simulink model "hx_sim"  (R2017b)
settings: Solver=ode23tb  StartTime=0.0  StopTime=tEndSimul  MaxStep=0.1  RelTol=5e-6
values from neighbouring files (symbols this model uses):
  dnDt_in = 1e-2    (= 0.01)    [hx.m]
  dnDt_out_liq = 1e-2    (= 0.01)    [hx.m]
  dnDt_out_vap = 1e-2    (= 0.01)    [hx.m]
  fluid = nh3_v4    [hx.m]
  Nhx_init = 100    [hx.m]
  q = 1e2    (= 100)    [hx.m]
  T_dnDt_in_C = 50    [hx.m]
  tEnd_dnDt_in = tStart_dnDt_in + 10 * c.min_to_sec    [hx.m]
  tEnd_dnDt_out_liq = tStart_dnDt_out_liq + 10 * c.min_to_sec    [hx.m]
  tEnd_dnDt_out_vap = tStart_dnDt_out_vap + 10 * c.min_to_sec    [hx.m]
  tEnd_q = tStart_q + 10 * c.min_to_sec    [hx.m]
  Thx_init = c.C_to_K(25)    [hx.m]
  tStart_dnDt_in = tEnd_q + 10 * c.min_to_sec    [hx.m]
  tStart_dnDt_out_liq = tEnd_dnDt_out_vap + 10 * c.min_to_sec    [hx.m]
  tStart_dnDt_out_vap = tEnd_dnDt_in + 10 * c.min_to_sec    [hx.m]
  tStart_q = 5 * c.min_to_sec    [hx.m]
  Vhx = 0.01    [hx.m]
libraries: thermochemical x20
settings Model: Creator=ferru  LastModifiedBy=fferrucc
settings SolverCC: AlgebraicLoopSolver=LineSearch

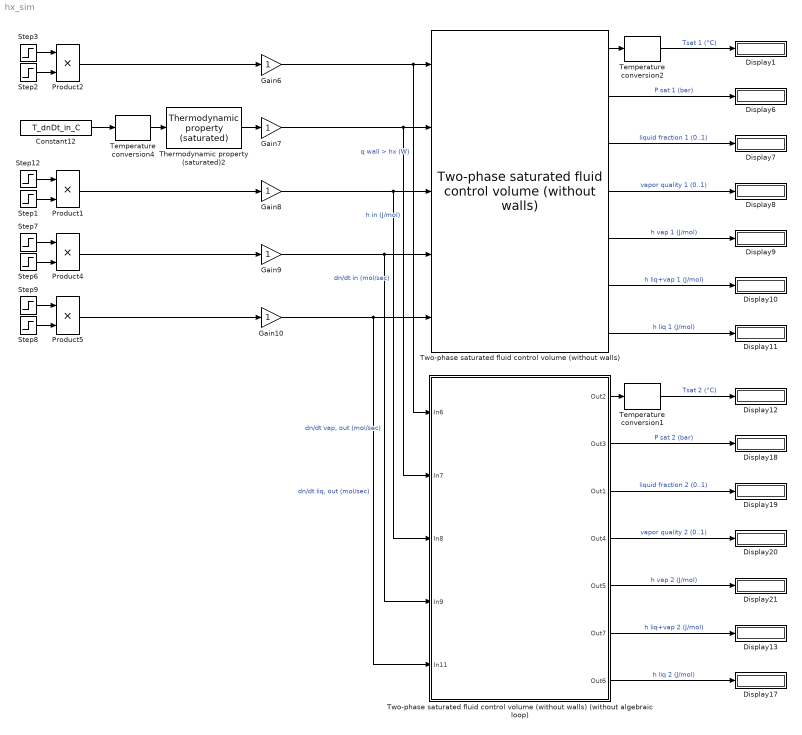
== system hx_sim ==
  Constant12 : Constant  Value=T_dnDt_in_C
  Display{1,6..13,17..21} (14 alike) : Display
  Gain{6..10} (5 alike) : Gain
  Product{1..2,4..5} (4 alike) : Product
  Step1 : Step  Time=tEnd_dnDt_in  Before=1  After=0  SampleTime=0
  Step12 : Step  Time=tStart_dnDt_in  After=dnDt_in  SampleTime=0
  Step2 : Step  Time=tEnd_q  Before=1  After=0  SampleTime=0
  Step3 : Step  Time=tStart_q  After=q  SampleTime=0
  Step6 : Step  Time=tEnd_dnDt_out_vap  Before=1  After=0  SampleTime=0
  Step7 : Step  Time=tStart_dnDt_out_vap  After=dnDt_out_vap  SampleTime=0
  Step8 : Step  Time=tEnd_dnDt_out_liq  Before=1  After=0  SampleTime=0
  Step9 : Step  Time=tStart_dnDt_out_liq  After=dnDt_out_liq  SampleTime=0
  Temperature conversion1 : thermochemical/Conversions/Temperature conversion  sel=K --> °C
      settings: SourceProductName=@ Thermochemical
  Temperature conversion2 : thermochemical/Conversions/Temperature conversion  sel=K --> °C
      settings: SourceProductName=@ Thermochemical
  Temperature conversion4 : thermochemical/Conversions/Temperature conversion  sel=°C --> K
      settings: SourceProductName=@ Thermochemical
  Thermodynamic property (saturated)2 : thermochemical/Thermodynamic fluid properties/Thermodynamic  property (saturated)  sel=h(T) vap. (J/mol)  fluid=fluid  lookup1D_BreakPoint1=fluid.sat.T  lookup1D_Data=fluid.sat.vap.h_molar
      settings: SourceProductName=@ Thermochemical
  Two-phase saturated fluid control volume (without walls) : thermochemical/Control volumes/Two-phase saturated fluid control volume (without walls)  N_init=Nhx_init  T_init=Thx_init  fluid=fluid  V=Vhx
      settings: SourceProductName=@ Thermochemical
  Two-phase saturated fluid control volume (without walls) (without algebraic loop) : Subsystem  AncestorBlock=|  mask(volume_control_saturated){N_init=Nhx_init, T_init=Thx_init, fluid=fluid, V=Vhx}
      | thermochemical/Control volumes/Two-phase saturated fluid
      | control volume (without walls)
      | (without algebraic loop)
      mask prompts: N_init "Initial number of mols inside the control volume (mol)"; T_init "Fluid initial temperature (K)"; fluid "Fluid (structure data type)"; V "Volume (m3)"
      mask help:
      | This block models a volume control that contains a fluid always in its saturation state.
      |
      | The model can work as a condenser or as an evaporator:
      | • Condenser: connect the output 'h liq (J/mol)' to the input 'h out (sat) (J/mol)'
      | • Evaporator: connect the output 'h vap (J/mol)' to the input 'h out (sat) (J/mol)'
      |
      | The ratio between the two phases is given by two outputs:
      | 1) volumetric liquid fraction: liquid volume/total volume (0..1)
      | 2) vapor quality (e.g. zero: 100% liquid, one: 100% vapor).
      |
      | Note 2: the model is not prepared to work in the non-saturation state of the fluid (e.g. superheated gas or supercooled liquid). This means that both the liquid fraction and the vapor quality are strictly constrained in the (0..1) open range. The simulation will stop if these constrains are violated.
      mask init:
      | c = conversion_factors();
      mask DialogControl Container3 Prompt: Initial state
      mask DialogControl Container4 Prompt: Other parameters
  wires:
  Step12/1 -> Product1/1
  Step1/1 -> Product1/2
  Constant12/1 -> Temperature conversion4/1
  Temperature conversion4/1 -> Thermodynamic property (saturated)2/1
  Temperature conversion2/1 -> Display1/1  "Tsat 1 (°C)"
  Two-phase saturated fluid control volume (without walls)/1 -> Temperature conversion2/1
  Gain6/1 -> Two-phase saturated fluid control volume (without walls) (without algebraic loop)/1(In6), Two-phase saturated fluid control volume (without walls)/1  "q wall > hx (W)"
  Gain7/1 -> Two-phase saturated fluid control volume (without walls) (without algebraic loop)/2(In7), Two-phase saturated fluid control volume (without walls)/2  "h in (J/mol)"
  Gain8/1 -> Two-phase saturated fluid control volume (without walls) (without algebraic loop)/3(In8), Two-phase saturated fluid control volume (without walls)/3  "dn/dt in (mol/sec)"
  Gain9/1 -> Two-phase saturated fluid control volume (without walls) (without algebraic loop)/4(In9), Two-phase saturated fluid control volume (without walls)/4  "dn/dt vap, out (mol/sec)"
  Gain10/1 -> Two-phase saturated fluid control volume (without walls) (without algebraic loop)/5(In11), Two-phase saturated fluid control volume (without walls)/5  "dn/dt liq, out (mol/sec)"
  Two-phase saturated fluid control volume (without walls)/2 -> Display6/1  "P sat 1 (bar)"
  Two-phase saturated fluid control volume (without walls)/3 -> Display7/1  "liquid fraction 1 (0..1)"
  Two-phase saturated fluid control volume (without walls)/4 -> Display8/1  "vapor quality 1 (0..1)"
  Two-phase saturated fluid control volume (without walls)/5 -> Display9/1  "h vap 1 (J/mol)"
  Two-phase saturated fluid control volume (without walls)/6 -> Display10/1  "h liq+vap 1 (J/mol)"
  Two-phase saturated fluid control volume (without walls)/7 -> Display11/1  "h liq 1 (J/mol)"
  Two-phase saturated fluid control volume (without walls) (without algebraic loop)/7(Out6) -> Display17/1  "h liq 2 (J/mol)"
  Two-phase saturated fluid control volume (without walls) (without algebraic loop)/6(Out7) -> Display13/1  "h liq+vap 2 (J/mol)"
  Two-phase saturated fluid control volume (without walls) (without algebraic loop)/5(Out5) -> Display21/1  "h vap 2 (J/mol)"
  Two-phase saturated fluid control volume (without walls) (without algebraic loop)/4(Out4) -> Display20/1  "vapor quality 2 (0..1)"
  Two-phase saturated fluid control volume (without walls) (without algebraic loop)/3(Out1) -> Display19/1  "liquid fraction 2 (0..1)"
  Two-phase saturated fluid control volume (without walls) (without algebraic loop)/2(Out3) -> Display18/1  "P sat 2 (bar)"
  Two-phase saturated fluid control volume (without walls) (without algebraic loop)/1(Out2) -> Temperature conversion1/1
  Temperature conversion1/1 -> Display12/1  "Tsat 2 (°C)"
  Step2/1 -> Product2/2
  Step3/1 -> Product2/1
  Product2/1 -> Gain6/1
  Thermodynamic property (saturated)2/1 -> Gain7/1
  Product1/1 -> Gain8/1
  Product4/1 -> Gain9/1
  Step6/1 -> Product4/2
  Step7/1 -> Product4/1
  Step9/1 -> Product5/1
  Step8/1 -> Product5/2
  Product5/1 -> Gain10/1

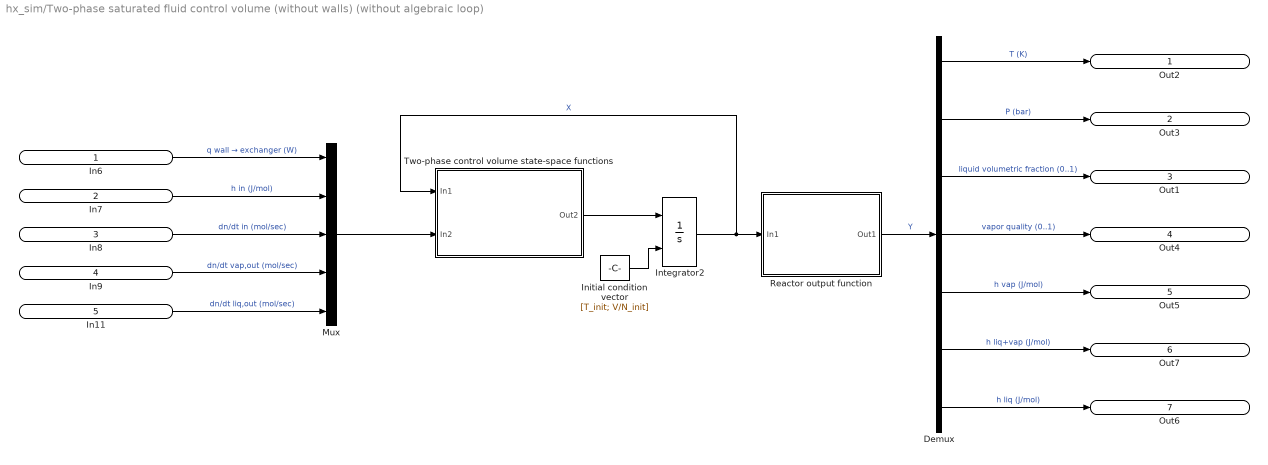
== system hx_sim/Two-phase saturated fluid control volume (without walls) (without algebraic loop) ==
  In6 : Inport
  In7 : Inport  Port=2
  In8 : Inport  Port=3
  In9 : Inport  Port=4
  In11 : Inport  Port=5
  Demux : Demux  Outputs=7
  Initial condition vector : Constant  Value=[T_init; V/N_init]
  Integrator2 : Integrator  InitialConditionSource=external
  Mux : Mux  Inputs=5
  Reactor output function : Subsystem
  Two-phase control volume state-space functions : Subsystem
  Out2 : Outport
  Out3 : Outport  Port=2
  Out1 : Outport  Port=3
  Out4 : Outport  Port=4
  Out5 : Outport  Port=5
  Out7 : Outport  Port=6
  Out6 : Outport  Port=7
  wires:
  Integrator2/1 -> Two-phase control volume state-space functions/1(In1), Reactor output function/1(In1)  "X"
  Initial condition vector/1 -> Integrator2/2
  Two-phase control volume state-space functions/1(Out2) -> Integrator2/1
  Mux/1 -> Two-phase control volume state-space functions/2(In2)
  Reactor output function/1(Out1) -> Demux/1  "Y"
  Demux/7 -> Out6/1  "h liq (J/mol)"
  Demux/2 -> Out3/1  "P (bar)"
  Demux/6 -> Out7/1  "h liq+vap (J/mol)"
  Demux/5 -> Out5/1  "h vap (J/mol)"
  Demux/4 -> Out4/1  "vapor quality (0..1)"
  Demux/1 -> Out2/1  "T (K)"
  Demux/3 -> Out1/1  "liquid volumetric fraction (0..1)"
  In6/1 -> Mux/1  "q wall → exchanger (W)"
  In11/1 -> Mux/5  "dn/dt liq,out (mol/sec)"
  In8/1 -> Mux/3  "dn/dt in (mol/sec)"
  In7/1 -> Mux/2  "h in (J/mol)"
  In9/1 -> Mux/4  "dn/dt vap,out (mol/sec)"

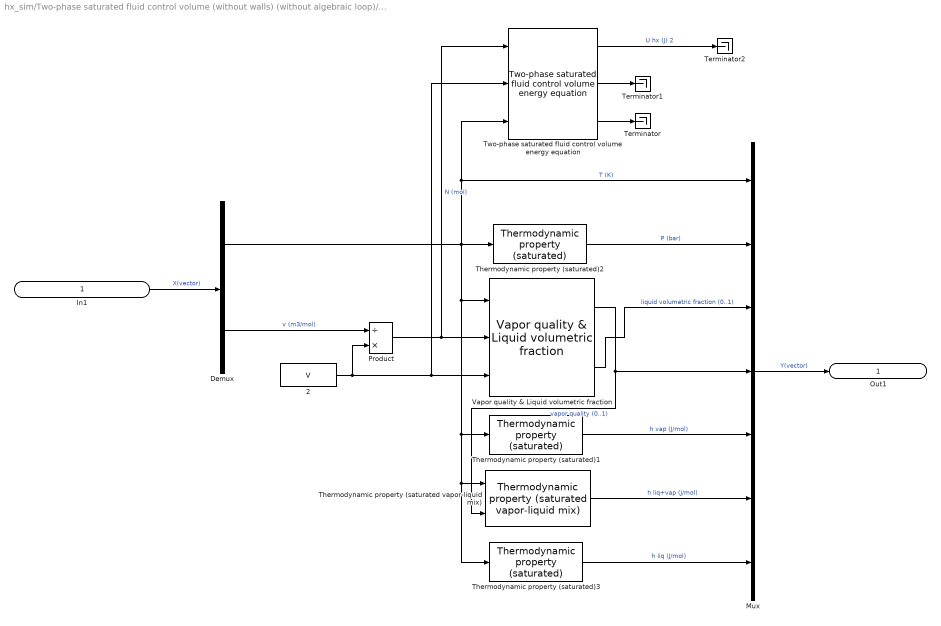
== system hx_sim/Two-phase saturated fluid control volume (without walls) (without algebraic loop)/Reactor output function ==
  In1 : Inport
  2 : Constant  Value=V
  Demux : Demux  Outputs=2
  Mux : Mux  Inputs=7
  Product : Product  Inputs=/*
  Terminator : Terminator
  Terminator1 : Terminator
  Terminator2 : Terminator
  Thermodynamic property (saturated)1 : thermochemical/Thermodynamic fluid properties/Thermodynamic  property (saturated)  sel=h(T) vap. (J/mol)  fluid=fluid  lookup1D_BreakPoint1=fluid.sat.T  lookup1D_Data=fluid.sat.vap.h_molar
      settings: SourceProductName=@ Thermochemical
  Thermodynamic property (saturated)2 : thermochemical/Thermodynamic fluid properties/Thermodynamic  property (saturated)  sel=P(T) (bar)  fluid=fluid  lookup1D_BreakPoint1=fluid.sat.T  lookup1D_Data=fluid.sat.Psat
      settings: SourceProductName=@ Thermochemical
  Thermodynamic property (saturated)3 : thermochemical/Thermodynamic fluid properties/Thermodynamic  property (saturated)  sel=h(T) liq. (J/mol)  fluid=fluid  lookup1D_BreakPoint1=fluid.sat.T  lookup1D_Data=fluid.sat.liq.h_molar
      settings: SourceProductName=@ Thermochemical
  Thermodynamic property (saturated vapor-liquid mix) : thermochemical/Thermodynamic fluid properties/Thermodynamic property  (saturated vapor-liquid mix)  sel=h(T) (J/mol)  fluid=fluid  lookup1D_BreakPoint=0  lookup1D_Data1=fluid.sat.liq.h_molar  lookup1D_Data2=fluid.sat.vap.h_molar
      settings: SourceProductName=@ Thermochemical
  Two-phase saturated fluid control volume energy equation : thermochemical/Control volumes/Two-phase saturated fluid control volume energy equation  fluid=fluid
      settings: SourceProductName=@ Thermochemical
  Vapor quality & Liquid volumetric fraction : thermochemical/Thermodynamic fluid properties/Vapor quality & Liquid  volumetric fraction  fluid=fluid
      settings: SourceProductName=@ Thermochemical
  Out1 : Outport
  wires:
  Demux/1 -> Thermodynamic property (saturated)3/1, Thermodynamic property (saturated vapor-liquid mix)/1, Thermodynamic property (saturated)1/1, Vapor quality & Liquid volumetric fraction/1, Two-phase saturated fluid control volume energy equation/3, Mux/1, Thermodynamic property (saturated)2/1  "T (K)"
  Demux/2 -> Product/1  "v (m3/mol)"
  Mux/1 -> Out1/1  "Y(vector)"
  In1/1 -> Demux/1  "X(vector)"
  Vapor quality & Liquid volumetric fraction/1 -> Thermodynamic property (saturated vapor-liquid mix)/2, Mux/4  "vapor quality (0..1)"
  Thermodynamic property (saturated)1/1 -> Mux/5  "h vap (J/mol)"
  Vapor quality & Liquid volumetric fraction/2 -> Mux/3  "liquid volumetric fraction (0..1)"
  Thermodynamic property (saturated vapor-liquid mix)/1 -> Mux/6  "h liq+vap (J/mol)"
  Thermodynamic property (saturated)2/1 -> Mux/2  "P (bar)"
  Thermodynamic property (saturated)3/1 -> Mux/7  "h liq (J/mol)"
  Product/1 -> Vapor quality & Liquid volumetric fraction/2, Two-phase saturated fluid control volume energy equation/1  "N (mol)"
  2/1 -> Two-phase saturated fluid control volume energy equation/2, Vapor quality & Liquid volumetric fraction/3, Product/2
  Two-phase saturated fluid control volume energy equation/3 -> Terminator/1
  Two-phase saturated fluid control volume energy equation/2 -> Terminator1/1
  Two-phase saturated fluid control volume energy equation/1 -> Terminator2/1  "U hx (J) 2"

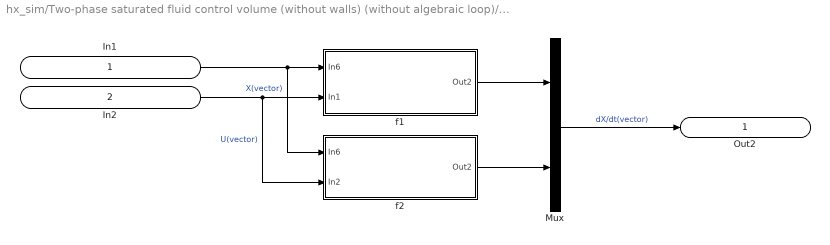
== system hx_sim/Two-phase saturated fluid control volume (without walls) (without algebraic loop)/Two-phase control volume state-space functions ==
  In1 : Inport
  In2 : Inport  Port=2
  Mux : Mux  Inputs=2
  f1 : Subsystem
  f2 : Subsystem
  Out2 : Outport
  wires:
  In2/1 -> f2/2(In2), f1/2(In1)  "U(vector)"
  In1/1 -> f2/1(In6), f1/1(In6)  "X(vector)"
  Mux/1 -> Out2/1  "dX/dt(vector)"
  f1/1(Out2) -> Mux/1
  f2/1(Out2) -> Mux/2

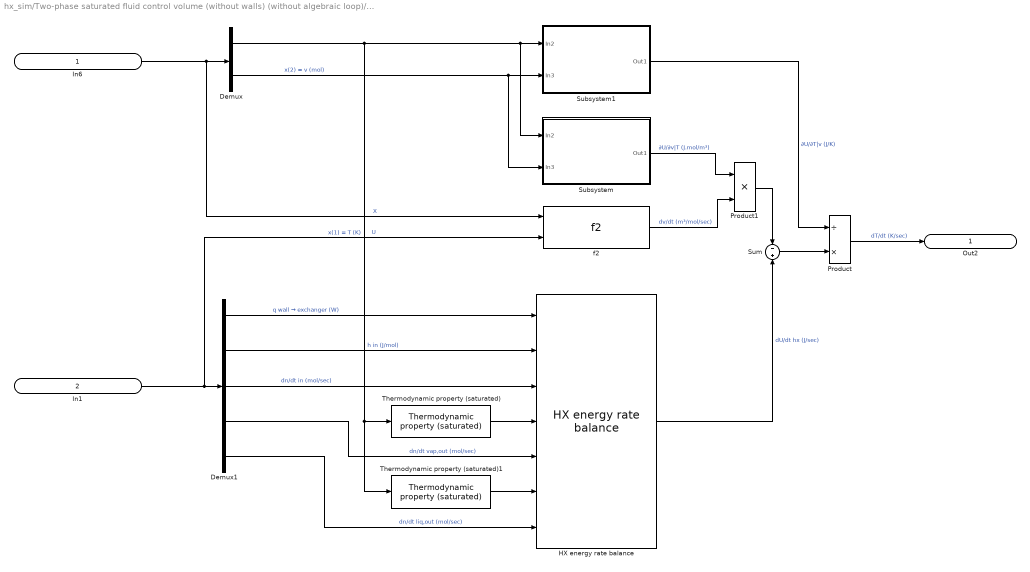
== system hx_sim/Two-phase saturated fluid control volume (without walls) (without algebraic loop)/Two-phase control volume state-space functions/f1 ==
  In6 : Inport
  In1 : Inport  Port=2
  Demux : Demux  Outputs=2
  Demux1 : Demux  Outputs=5
  HX energy rate balance : thermochemical/Control volumes/Two-phase saturated fluid control volume (without walls)/Internal energy differential equation/HX energy rate balance
      settings: SourceProductName=@ Thermochemical
  Product : Product  Inputs=/*
  Product1 : Product  Inputs=**
  Subsystem : Subsystem
  Subsystem1 : Subsystem
  Sum : Sum  Inputs=-+
  Thermodynamic property (saturated) : thermochemical/Thermodynamic fluid properties/Thermodynamic  property (saturated)  sel=h(T) vap. (J/mol)  fluid=fluid  lookup1D_BreakPoint1=fluid.sat.T  lookup1D_Data=fluid.sat.vap.h_molar
      settings: SourceProductName=@ Thermochemical
  Thermodynamic property (saturated)1 : thermochemical/Thermodynamic fluid properties/Thermodynamic  property (saturated)  sel=h(T) liq. (J/mol)  fluid=fluid  lookup1D_BreakPoint1=fluid.sat.T  lookup1D_Data=fluid.sat.liq.h_molar
      settings: SourceProductName=@ Thermochemical
  f2 : thermochemical/Control volumes/Two-phase saturated fluid control volume (without walls) (without algebraic loop)/Two-phase control volume state-space functions/f2
      settings: SourceProductName=@ Thermochemical
  Out2 : Outport
  wires:
  Product/1 -> Out2/1  "dT/dt (K/sec)"
  Demux/2 -> Subsystem/2(In3), Subsystem1/2(In3)  "x(2) = v (mol)"
  In6/1 -> f2/1, Demux/1  "X"
  In1/1 -> f2/2, Demux1/1  "U"
  Demux/1 -> Thermodynamic property (saturated)1/1, Thermodynamic property (saturated)/1, Subsystem/1(In2), Subsystem1/1(In2)  "x(1) = T (K)"
  HX energy rate balance/1 -> Sum/2  "dU/dt hx (J/sec)"
  Subsystem/1(Out1) -> Product1/1  "∂U/∂v|T (J.mol/m³)"
  Subsystem1/1(Out1) -> Product/1  "∂U/∂T|v (J/K)"
  f2/1 -> Product1/2  "dv/dt (m³/mol/sec)"
  Sum/1 -> Product/2
  Product1/1 -> Sum/1
  Demux1/1 -> HX energy rate balance/1  "q wall → exchanger (W)"
  Demux1/3 -> HX energy rate balance/3  "dn/dt in (mol/sec)"
  Demux1/4 -> HX energy rate balance/5  "dn/dt vap,out (mol/sec)"
  Demux1/2 -> HX energy rate balance/2  "h in (J/mol)"
  Demux1/5 -> HX energy rate balance/7  "dn/dt liq,out (mol/sec)"
  Thermodynamic property (saturated)/1 -> HX energy rate balance/4
  Thermodynamic property (saturated)1/1 -> HX energy rate balance/6

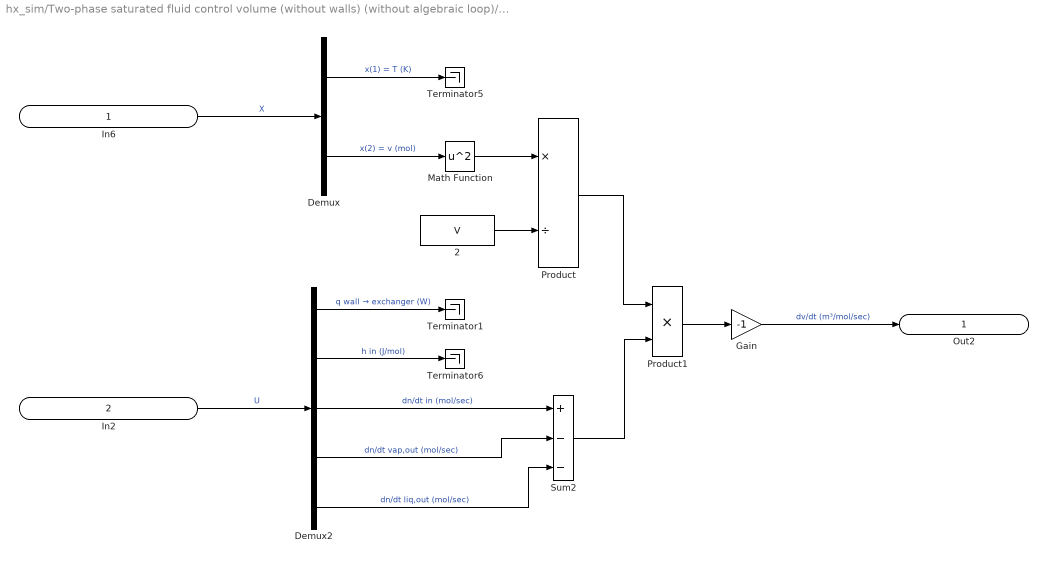
== system hx_sim/Two-phase saturated fluid control volume (without walls) (without algebraic loop)/Two-phase control volume state-space functions/f2 ==
  In6 : Inport
  In2 : Inport  Port=2
  2 : Constant  Value=V
  Demux : Demux  Outputs=2
  Demux2 : Demux  Outputs=5
  Gain : Gain  Gain=-1
  Math Function : Math  Operator=square  SaturateOnIntegerOverflow=on
  Product : Product  Inputs=*/
  Product1 : Product  Inputs=**
  Sum2 : Sum  Inputs=+--
  Terminator1 : Terminator
  Terminator5 : Terminator
  Terminator6 : Terminator
  Out2 : Outport
  wires:
  Demux/1 -> Terminator5/1  "x(1) = T (K)"
  In6/1 -> Demux/1  "X"
  Product1/1 -> Gain/1
  Demux/2 -> Math Function/1  "x(2) = v (mol)"
  Sum2/1 -> Product1/2
  Math Function/1 -> Product/1
  2/1 -> Product/2
  Product/1 -> Product1/1
  Demux2/2 -> Terminator6/1  "h in (J/mol)"
  Demux2/3 -> Sum2/1  "dn/dt in (mol/sec)"
  Demux2/1 -> Terminator1/1  "q wall → exchanger (W)"
  Demux2/5 -> Sum2/3  "dn/dt liq,out (mol/sec)"
  Demux2/4 -> Sum2/2  "dn/dt vap,out (mol/sec)"
  In2/1 -> Demux2/1  "U"
  Gain/1 -> Out2/1  "dv/dt (m³/mol/sec)"

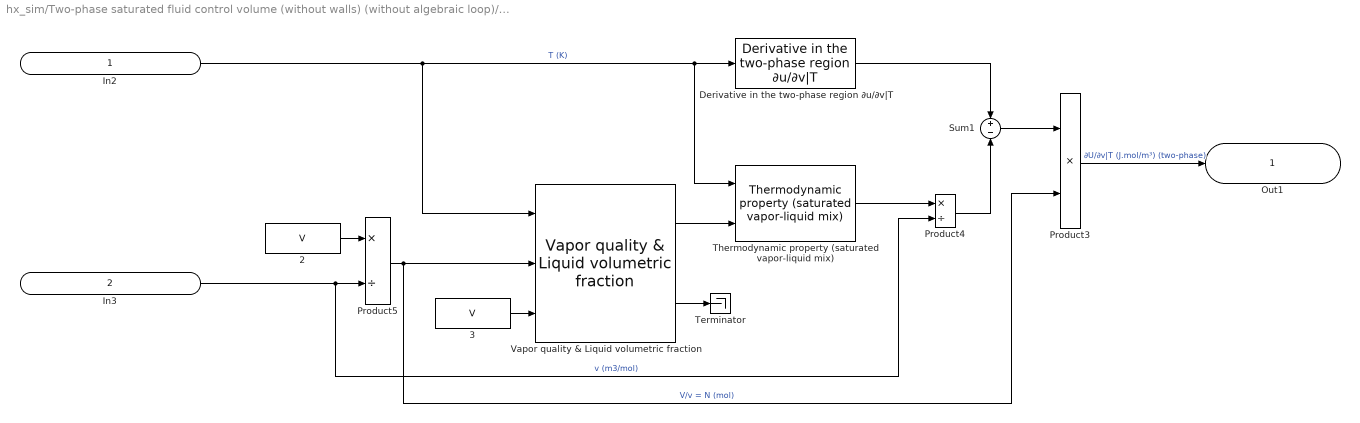
== system hx_sim/Two-phase saturated fluid control volume (without walls) (without algebraic loop)/Two-phase control volume state-space functions/f1/Subsystem ==
  In2 : Inport
  In3 : Inport  Port=2
  2 : Constant  Value=V
  3 : Constant  Value=V
  Derivative in the two-phase region ∂u/∂v|T : thermochemical/Thermodynamic fluid properties/Derivative in the two-phase region ∂u//∂v|T  fluid=fluid
      settings: SourceProductName=@ Thermochemical
  Product3 : Product  Inputs=**
  Product4 : Product  Inputs=*/
  Product5 : Product  Inputs=*/
  Sum1 : Sum  Inputs=+-
  Terminator : Terminator
  Thermodynamic property (saturated vapor-liquid mix) : thermochemical/Thermodynamic fluid properties/Thermodynamic property  (saturated vapor-liquid mix)  sel=u(T) (J/mol)  fluid=fluid  lookup1D_BreakPoint=0  lookup1D_Data1=fluid.sat.liq.u_molar  lookup1D_Data2=fluid.sat.vap.u_molar
      settings: SourceProductName=@ Thermochemical
  Vapor quality & Liquid volumetric fraction : thermochemical/Thermodynamic fluid properties/Vapor quality & Liquid  volumetric fraction  fluid=fluid
      settings: SourceProductName=@ Thermochemical
  Out1 : Outport
  wires:
  Product4/1 -> Sum1/2
  Sum1/1 -> Product3/1
  Derivative in the two-phase region ∂u/∂v|T/1 -> Sum1/1
  3/1 -> Vapor quality & Liquid volumetric fraction/3
  2/1 -> Product5/1
  Vapor quality & Liquid volumetric fraction/1 -> Thermodynamic property (saturated vapor-liquid mix)/2
  Product3/1 -> Out1/1  "∂U/∂v|T (J.mol/m³) (two-phase)"
  Product5/1 -> Product3/2, Vapor quality & Liquid volumetric fraction/2  "V/v = N (mol)"
  In3/1 -> Product4/2, Product5/2  "v (m3/mol)"
  In2/1 -> Derivative in the two-phase region ∂u/∂v|T/1, Thermodynamic property (saturated vapor-liquid mix)/1, Vapor quality & Liquid volumetric fraction/1  "T (K)"
  Thermodynamic property (saturated vapor-liquid mix)/1 -> Product4/1
  Vapor quality & Liquid volumetric fraction/2 -> Terminator/1

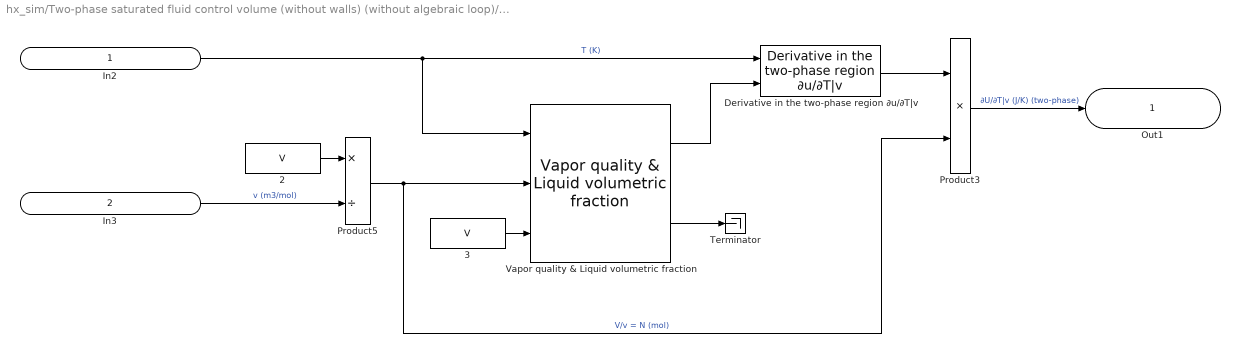
== system hx_sim/Two-phase saturated fluid control volume (without walls) (without algebraic loop)/Two-phase control volume state-space functions/f1/Subsystem1 ==
  In2 : Inport
  In3 : Inport  Port=2
  2 : Constant  Value=V
  3 : Constant  Value=V
  Derivative in the two-phase region ∂u/∂T|v : thermochemical/Thermodynamic fluid properties/Derivative in the two-phase region ∂u//∂T|v  fluid=fluid
      settings: SourceProductName=@ Thermochemical
  Product3 : Product  Inputs=**
  Product5 : Product  Inputs=*/
  Terminator : Terminator
  Vapor quality & Liquid volumetric fraction : thermochemical/Thermodynamic fluid properties/Vapor quality & Liquid  volumetric fraction  fluid=fluid
      settings: SourceProductName=@ Thermochemical
  Out1 : Outport
  wires:
  Vapor quality & Liquid volumetric fraction/2 -> Terminator/1
  In2/1 -> Derivative in the two-phase region ∂u/∂T|v/1, Vapor quality & Liquid volumetric fraction/1  "T (K)"
  In3/1 -> Product5/2  "v (m3/mol)"
  Product5/1 -> Product3/2, Vapor quality & Liquid volumetric fraction/2  "V/v = N (mol)"
  Product3/1 -> Out1/1  "∂U/∂T|v (J/K) (two-phase)"
  Vapor quality & Liquid volumetric fraction/1 -> Derivative in the two-phase region ∂u/∂T|v/2
  2/1 -> Product5/1
  3/1 -> Vapor quality & Liquid volumetric fraction/3
  Derivative in the two-phase region ∂u/∂T|v/1 -> Product3/1
